simulink model "Active_Suspension_LQR"  (R2023a)
settings: Solver=VariableStepAuto  StartTime=0.0  StopTime=10  RelTol=1e-3
settings Model: Creator=nanda  LastModifiedBy=nanda

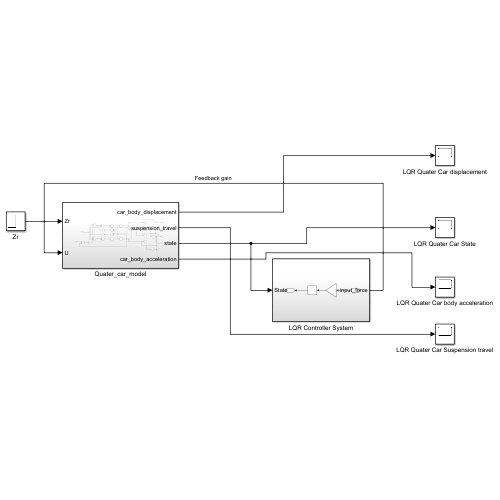
[thumbnail: Simulink's stored preview of the top-level diagram]
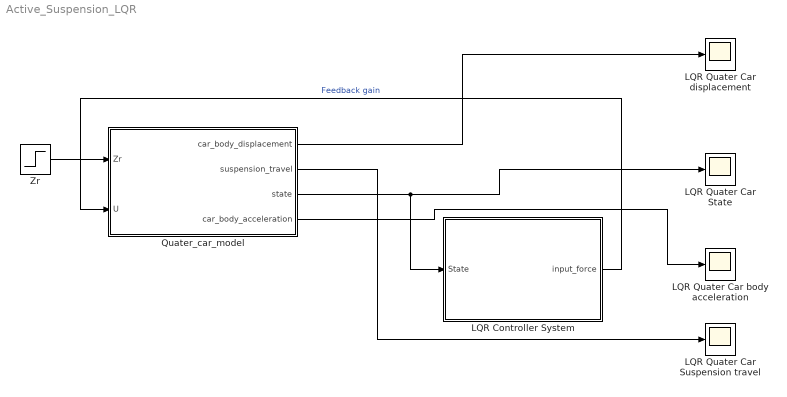
== system Active_Suspension_LQR ==
  LQR Controller System : Subsystem
  LQR Quater Car State : Scope
  LQR Quater Car Suspension travel : Scope
  LQR Quater Car body acceleration : Scope
  LQR Quater Car displacement : Scope
  Quater_car_model : Subsystem
  Zr : Step  After=0.5  SampleTime=0
  wires:
  Quater_car_model/4(car_body_acceleration) -> LQR Quater Car body acceleration/1
  Quater_car_model/1(car_body_displacement) -> LQR Quater Car displacement/1
  Quater_car_model/2(suspension_travel) -> LQR Quater Car Suspension travel/1
  LQR Controller System/1(input_force) -> Quater_car_model/2(U)  "Feedback gain"
  Zr/1 -> Quater_car_model/1(Zr)
  Quater_car_model/3(state) -> LQR Quater Car State/1, LQR Controller System/1(State)

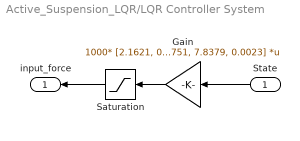
== system Active_Suspension_LQR/LQR Controller System ==
  State : Inport
  Gain : Gain  Gain=1000* [2.1621, 0.7751, 7.8379, 0.0023]  Multiplication=Matrix(K*u)
  Saturation : Saturate  UpperLimit=46730  LowerLimit=-46730
  input_force : Outport
  wires:
  Saturation/1 -> input_force/1
  Gain/1 -> Saturation/1
  State/1 -> Gain/1

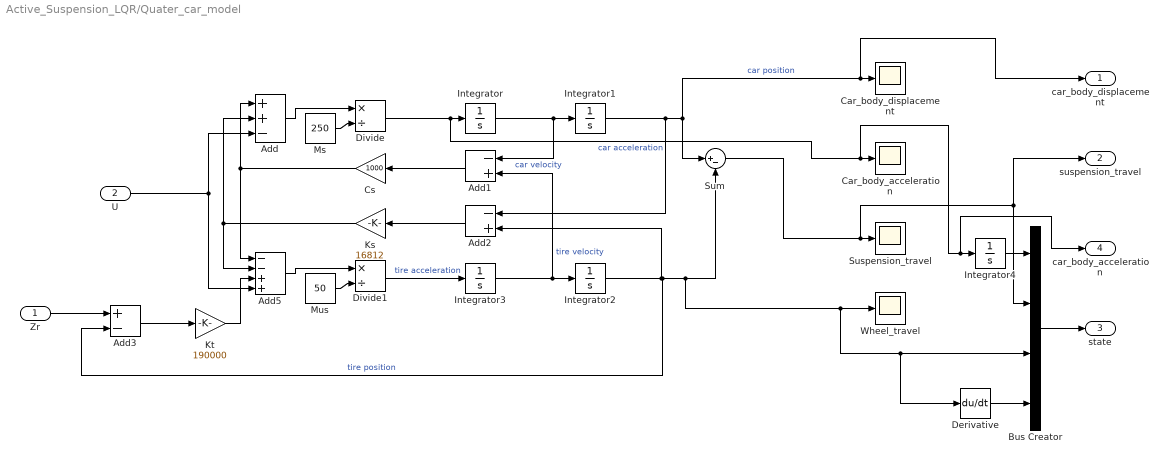
== system Active_Suspension_LQR/Quater_car_model ==
  Zr : Inport
  U : Inport  Port=2
  Add : Sum  Inputs=++-
  Add1 : Sum  Inputs=-+
  Add2 : Sum  Inputs=-+
  Add3 : Sum  Inputs=+-
  Add5 : Sum  Inputs=--++
  Bus Creator : BusCreator  Inputs=4
  Car_body_acceleration : Scope
  Car_body_displacement : Scope
  Cs : Gain  Gain=1000
  Derivative : Derivative
  Divide : Product  Inputs=*/
  Divide1 : Product  Inputs=*/
  Integrator{,1..4} (5 alike) : Integrator
  Ks : Gain  Gain=16812
  Kt : Gain  Gain=190000
  Ms : Constant  Value=250
  Mus : Constant  Value=50
  Sum : Sum  Inputs=|+-
  Suspension_travel : Scope
  Wheel_travel : Scope
  car_body_displacement : Outport
  suspension_travel : Outport  Port=2
  state : Outport  Port=3
  car_body_acceleration : Outport  Port=4
  wires:
  Derivative/1 -> Bus Creator/4
  Integrator4/1 -> Bus Creator/1
  Integrator1/1 -> car_body_displacement/1, Car_body_displacement/1, Sum/1, Add2/1  "car position"
  Add1/1 -> Cs/1
  Divide1/1 -> Integrator3/1  "tire acceleration"
  Mus/1 -> Divide1/2
  Integrator3/1 -> Integrator2/1, Add1/2  "tire velocity"
  Sum/1 -> suspension_travel/1, Bus Creator/2, Suspension_travel/1
  Cs/1 -> Add/1, Add5/1
  Divide/1 -> car_body_acceleration/1, Integrator4/1, Car_body_acceleration/1, Integrator/1  "car acceleration"
  Kt/1 -> Add5/3
  Integrator2/1 -> Add3/2, Wheel_travel/1, Derivative/1, Bus Creator/3, Sum/2, Add2/2  "tire position"
  Integrator/1 -> Integrator1/1, Add1/1  "car velocity"
  Ks/1 -> Add5/2, Add/2
  Add2/1 -> Ks/1
  Add5/1 -> Divide1/1
  Add/1 -> Divide/1
  Ms/1 -> Divide/2
  Bus Creator/1 -> state/1
  U/1 -> Add/3, Add5/4
  Add3/1 -> Kt/1
  Zr/1 -> Add3/1
